simulink model "TP_Avion_Eleve_2018b"  (R2018b)
settings: Solver=VariableStepAuto  StartTime=0.0  StopTime=25  RelTol=1e-3
libraries: simulink x1
settings Model: Creator=xpess  LastModifiedBy=xpess

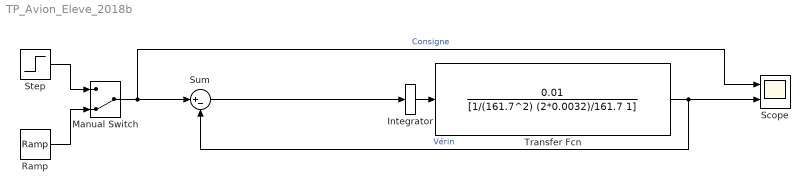
== system TP_Avion_Eleve_2018b ==
  Integrator : Integrator
  Manual Switch : ManualSwitch  CurrentSetting=0
  Ramp : simulink/Sources/Ramp  slope=1  start=0  InitialOutput=0
  Scope : Scope  NumInputPorts=2
  Step : Step  Time=0  SampleTime=0
  Sum : Sum  Inputs=|+-
  Transfer Fcn : TransferFcn  Numerator=[0.01]  Denominator=[1/(161.7^2) (2*0.0032)/161.7 1]
  wires:
  Step/1 -> Manual Switch/1
  Transfer Fcn/1 -> Scope/2, Sum/2  "Vérin"
  Integrator/1 -> Transfer Fcn/1
  Ramp/1 -> Manual Switch/2
  Manual Switch/1 -> Scope/1, Sum/1  "Consigne"
  Sum/1 -> Integrator/1
